simulink model "FOC_ADRC1"  (R2021b)
settings: Solver=ode3  StartTime=0.0  StopTime=0.6
InitFcn:
  | Ld=0.2e-3;
  | Lq=0.47e-3;
  | flux=0.062;
  | Rs=0.025;
  | b=1600;
libraries: simulink x2, spsDCVoltageSourceLib x1, spsPermanentMagnetSynchronousMachineLib x1, spsUniversalBridgeLib x1, spspowerguiLib x1
settings Model: SimulationMode=accelerator  Creator=lzy  LastModifiedBy=乐无安
settings SolverCC: AlgebraicLoopSolver=LineSearch
settings DebuggingCC: SFMachineParentedDataDiag=warning

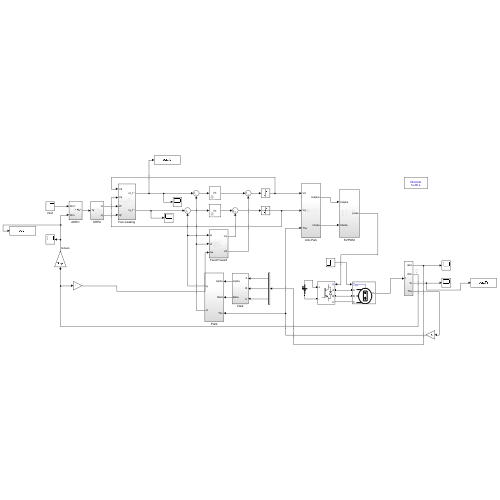
[thumbnail: Simulink's stored preview of the top-level diagram]
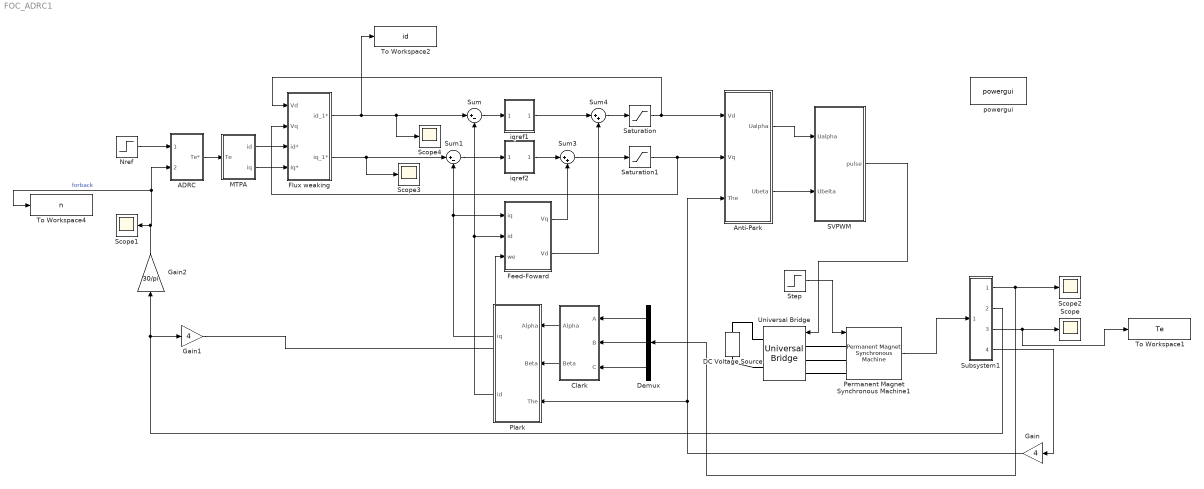
== system FOC_ADRC1 ==
  ADRC : Subsystem
  Anti-Park : Subsystem
  Clark : Subsystem
  DC Voltage Source : spsDCVoltageSourceLib/DC Voltage Source  Amplitude=192  Measurements=None
  Demux : Demux  Outputs=3
  Feed-Foward : Subsystem
  Flux weaking : Subsystem
  Gain : Gain  Gain=4
  Gain1 : Gain  Gain=4
  Gain2 : Gain  Gain=30/pi
  MTPA : Subsystem
  Nref : Step  Time=0.2  Before=3500  After=5500  SampleTime=0
  Permanent Magnet Synchronous Machine1 : spsPermanentMagnetSynchronousMachineLib/Permanent Magnet Synchronous Machine  NbPhases=3  FluxDistribution=Sinusoidal  RotorType=Salient-pole  MechanicalLoad=Torque Tm  PresetModel=No  ShowDetailedParameters=on  MeasurementBus=off  Resistance=0.029  Inductance=8.5e-3  dqInductances=[0.2e-3 0.47e-3]  La=0.015  MachineConstant=Flux linkage established by magnets (V.s)  Flux=0.062  VoltageCst=44.9822  TorqueCst=0.372  Flat=120  Mechanical=[1e-2 0 4]  PolePairs=3  InitialConditions=[0,0, 0,0]  InitialConditions5ph=[0 0 0 0 0 0]  RefAngle=Aligned with phase A axis (original Park)  IterativeDiscreteModel=Trapezoidal non iterative  TsBlock=-1  TsPowergui=0
  Plark : Subsystem
  SVPWM : Subsystem
  Saturation : Saturate  UpperLimit=192/1.732  LowerLimit=-192/1.732
  Saturation1 : Saturate  UpperLimit=192/1.732  LowerLimit=-192/1.732
  Scope{,1..4} (5 alike) : Scope
  Step : Step  Time=0.4  After=13  SampleTime=0
  Subsystem1 : Subsystem
  Sum : Sum  Inputs=|+-
  Sum1 : Sum  Inputs=|+-
  Sum3 : Sum  Inputs=|++
  Sum4 : Sum  Inputs=|++
  To Workspace1 : ToWorkspace  VariableName=Te  SampleTime=-1
      settings: Save2DSignal=2-D array (concatenate along first dimension)
  To Workspace2 : ToWorkspace  VariableName=id  SampleTime=-1
      settings: Save2DSignal=2-D array (concatenate along first dimension)
  To Workspace4 : ToWorkspace  VariableName=n  SampleTime=-1
      settings: Save2DSignal=2-D array (concatenate along first dimension)
  Universal Bridge : spsUniversalBridgeLib/Universal Bridge  Arms=3  SnubberResistance=1e5  SnubberCapacitance=inf  Device=IGBT / Diodes  Ron=1e-3  Lon=0  ForwardVoltages="[  0  0  ]"  ForwardVoltage=0  GTOparameters=[ 10e-6 , 20e-6 ]  IGBTparameters=[ 1e-6 , 2e-6 ]  Measurements=None  Measurements_2=None  converterType=Rectifier
  iqref1 : Subsystem  mask(PI Controller){I=60, P=40, sat=[-192/1.732,192/1.732]}
      mask prompts: I "Integral"; P "Proportional:"; sat "Minimum and maximum outputs:"
      mask init:
      | min=sat(1);max=sat(2);
      mask Display: disp('PI')
  iqref2 : Subsystem  mask(PI Controller){I=60, P=20, sat=[-192/1.732,192/1.732]}
      mask prompts: I "Integral"; P "Proportional:"; sat "Minimum and maximum outputs:"
      mask init:
      | min=sat(1);max=sat(2);
      mask Display: disp('PI')
  powergui : spspowerguiLib/powergui  Priority=1  SimulationMode=Discrete  SampleTime=10e-7  frequency=60  Iterations=50  frequencyindice=0  Pbase=100e6  ErrMax=1e-4  UnitsV=kV  UnitsW=MW  buscounter=0  FunctionMessages=off  echomessages=off  EnableUseOfTLC=off  CurrentSourceSwitches=off  DisableSnubberDevices=off  DisableRonSwitches=off  DisableVfSwitches=off  DisplayEquations=off  AutomaticDiscreteSolvers=off  SolverType=Tustin/Backward Euler (TBE)  Interpol=off  ExternalGateDelay=off  methode=off  Ts=100  x0status=blocks  SPID=on  SwTol=0  HookPort=off  NonlinearTolerance=1e-4  nMaxIteration=100  ContinueOnMaxIteration=off  RestoreLinks=warning  ResistiveCurrentMeasurement=off  Frange=[0:2:500]  Ylog=off  Xlog=on  ShowGrid=off  save=off  variable=ZData  structure=0  ZoomFFT=off  StartTime=0.0  cycles=1  DisplayStyle=1  fundamental=60  FreqAxis=off  MaxFrequency=1000  frequencyindicesteady=1  RmsSteady=1  display=off
  wires:
  Subsystem1/1(iabc) -> Scope2/1, Demux/1
  Sum/1 -> iqref1/1(In_1)
  Sum1/1 -> iqref2/1(In_1)
  Subsystem1/3(Te) -> To Workspace1/1, Scope/1
  Subsystem1/2(Wm) -> Gain1/1, Gain2/1
  Permanent Magnet Synchronous Machine1/1 -> Subsystem1/1(In1)
  Flux weaking/2(iq_1*) -> Scope3/1, Sum1/1
  Sum4/1 -> Saturation/1
  Sum3/1 -> Saturation1/1
  iqref2/1(Out_1) -> Sum3/1
  iqref1/1(Out_1) -> Sum4/1
  MTPA/1(id) -> Flux weaking/3(id*)
  Gain2/1 -> Scope1/1, To Workspace4/1, ADRC/2(Wm)  "forback"
  Step/1 -> Permanent Magnet Synchronous Machine1/1
  Clark/1(Alpha) -> Plark/1(Alpha)
  Demux/1 -> Clark/1(A)
  Demux/2 -> Clark/2(B)
  Demux/3 -> Clark/3(C)
  SVPWM/1(pulse) -> Universal Bridge/1
  ADRC/1(Te*) -> MTPA/1(Te)
  Anti-Park/1(Ualpha) -> SVPWM/1(Ualpha)
  Anti-Park/2(Ubeta) -> SVPWM/2(Ubelta)
  Subsystem1/4(The) -> Gain/1
  Clark/2(Beta) -> Plark/2(Beta)
  Plark/2(id) -> Feed-Foward/2(id), Sum/2
  Plark/1(iq) -> Feed-Foward/1(iq), Sum1/2
  Flux weaking/1(id_1*) -> To Workspace2/1, Scope4/1, Sum/1
  Gain1/1 -> Feed-Foward/3(we)
  Feed-Foward/1(Vq) -> Sum3/2
  Feed-Foward/2(Vd) -> Sum4/2
  Gain/1 -> Anti-Park/3(The), Plark/3(The)
  MTPA/2(iq) -> Flux weaking/4(Iq*)
  Nref/1 -> ADRC/1(Wm*)
  Saturation1/1 -> Flux weaking/2(Vq), Anti-Park/2(Vq)
  Saturation/1 -> Flux weaking/1(Vd), Anti-Park/1(Vd)
  connections:
  Universal Bridge/RConn1 -- DC Voltage Source/RConn1
  Universal Bridge/RConn2 -- DC Voltage Source/LConn1
  Universal Bridge/LConn3 -- Permanent Magnet Synchronous Machine1/LConn3
  Permanent Magnet Synchronous Machine1/LConn2 -- Universal Bridge/LConn2
  Permanent Magnet Synchronous Machine1/LConn1 -- Universal Bridge/LConn1

== system FOC_ADRC1/ADRC ==
  Wm* : Inport
  Wm : Inport  Port=2
  1/b : Gain  Gain=1/2000
  ESO : Subsystem
  Nlsef : Subsystem
  Saturation : Saturate  UpperLimit=72  LowerLimit=-72
  Sum : Sum  Inputs=|+-
  TD : Subsystem
  b : Gain  Gain=b
  Te* : Outport
  wires:
  Wm/1 -> ESO/2(Wm)
  Wm*/1 -> TD/1(Wm*)
  b/1 -> ESO/1(bu)
  TD/1(Z11) -> Nlsef/1(Z11)
  1/b/1 -> Sum/2
  Nlsef/1(u0) -> Sum/1
  Sum/1 -> Saturation/1, b/1
  Saturation/1 -> Te*/1
  ESO/2(Z21) -> Nlsef/2(Z21)
  ESO/1(Z22) -> 1/b/1

== system FOC_ADRC1/Anti-Park ==
  Vd : Inport
  Vq : Inport  Port=2
  The : Inport  Port=3
  Fcn : Fcn  Expr=cos(u[1])*u[2]-sin(u[1])*u[3]
  Fcn1 : Fcn  Expr=sin(u[1])*u[2]+cos(u[1])*u[3]
  Mux1 : Mux  Inputs=3
  Ualpha : Outport  VectorParamsAs1DForOutWhenUnconnected=off
  Ubeta : Outport  Port=2  VectorParamsAs1DForOutWhenUnconnected=off
  wires:
  Vd/1 -> Mux1/2
  The/1 -> Mux1/1
  Fcn1/1 -> Ubeta/1
  Vq/1 -> Mux1/3
  Fcn/1 -> Ualpha/1
  Mux1/1 -> Fcn/1, Fcn1/1

== system FOC_ADRC1/Clark ==
  A : Inport
  B : Inport  Port=2
  C : Inport  Port=3
  Mux : Mux  Inputs=3
  alpha : Fcn  Expr=(u(1)-0.5*(u(2)+u(3)))*2/3
  beta : Fcn  Expr=sqrt(3)/2*(u(2)-u(3))*2/3
  Alpha : Outport  VectorParamsAs1DForOutWhenUnconnected=off
  Beta : Outport  Port=2  VectorParamsAs1DForOutWhenUnconnected=off
  wires:
  B/1 -> Mux/2
  C/1 -> Mux/3
  beta/1 -> Beta/1
  A/1 -> Mux/1
  Mux/1 -> beta/1, alpha/1
  alpha/1 -> Alpha/1

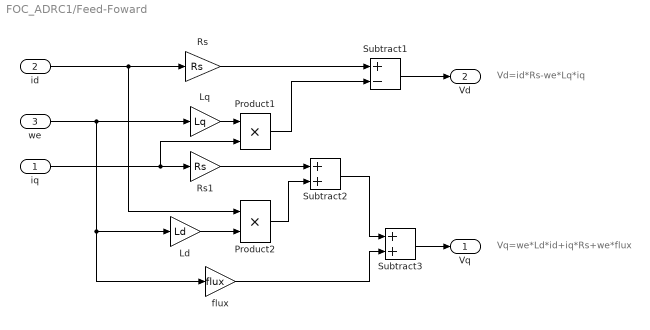
== system FOC_ADRC1/Feed-Foward ==
  note: Vd=id*Rs-we*Lq*iq
  note: Vq=we*Ld*id+iq*Rs+we*flux
  iq : Inport
  id : Inport  Port=2
  we : Inport  Port=3
  Ld : Gain  Gain=Ld
  Lq : Gain  Gain=Lq
  Product1 : Product  RndMeth=Zero
  Product2 : Product  RndMeth=Zero
  Rs : Gain  Gain=Rs
  Rs1 : Gain  Gain=Rs
  Subtract1 : Sum  Inputs=+-
  Subtract2 : Sum
  Subtract3 : Sum
  flux : Gain  Gain=flux
  Vq : Outport  VectorParamsAs1DForOutWhenUnconnected=off
  Vd : Outport  Port=2  VectorParamsAs1DForOutWhenUnconnected=off
  wires:
  Subtract2/1 -> Subtract3/1
  iq/1 -> Rs1/1, Product1/2
  we/1 -> Lq/1, Ld/1, flux/1
  flux/1 -> Subtract3/2
  Product2/1 -> Subtract2/2
  id/1 -> Rs/1, Product2/1
  Lq/1 -> Product1/1
  Product1/1 -> Subtract1/2
  Subtract1/1 -> Vd/1
  Rs/1 -> Subtract1/1
  Rs1/1 -> Subtract2/1
  Ld/1 -> Product2/2
  Subtract3/1 -> Vq/1

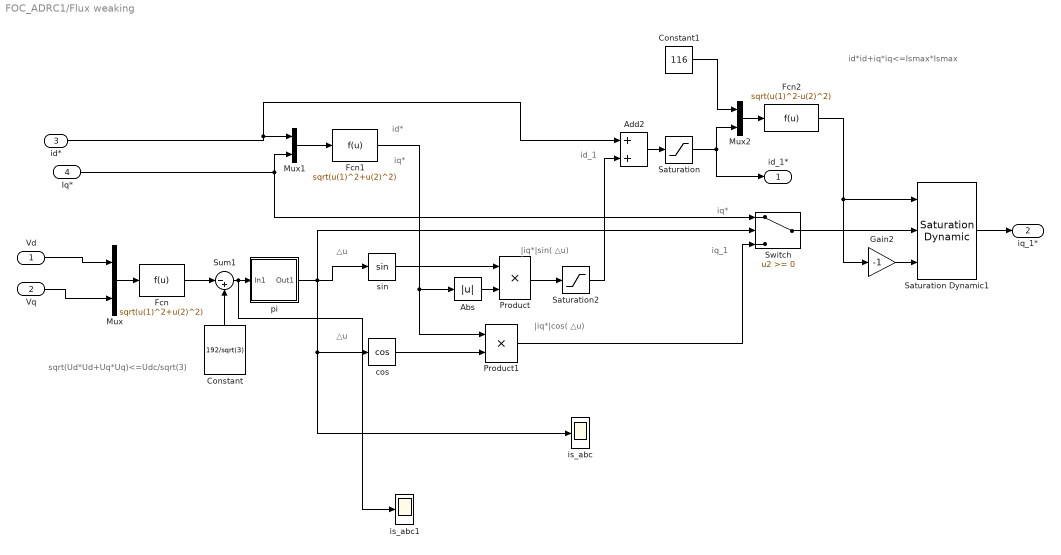
== system FOC_ADRC1/Flux weaking ==
  note: |iq*|cos( △u)
  note: iq*
  note: id*id+iq*iq<=Ismax*Ismax
  note: |iq*|sin( △u)
  note: sqrt(Ud*Ud+Uq*Uq)<=Udc/sqrt(3)
  note: id*
  note: △u
  note: △u
  note: iq*
  note: id_1
  note: iq_1
  Vd : Inport
  Vq : Inport  Port=2
  id* : Inport  Port=3
  Iq* : Inport  Port=4
  Abs : Abs
  Add2 : Sum  OutDataTypeStr=Inherit: Same as first input
  Constant : Constant  Value=192/sqrt(3)  SampleTime=-1
  Constant1 : Constant  Value=116  SampleTime=-1
  Fcn : Fcn  Expr=sqrt(u(1)^2+u(2)^2)
  Fcn1 : Fcn  Expr=sqrt(u(1)^2+u(2)^2)
  Fcn2 : Fcn  Expr=sqrt(u(1)^2-u(2)^2)
  Gain2 : Gain  Gain=-1
  Mux : Mux  Inputs=2
  Mux1 : Mux  Inputs=2
  Mux2 : Mux  Inputs=2
  Product : Product  RndMeth=Zero
  Product1 : Product  RndMeth=Zero
  Saturation : Saturate  UpperLimit=100  LowerLimit=-100
  Saturation Dynamic1 : simulink/Discontinuities/Saturation Dynamic  OutMin=[]  OutMax=[]  OutDataTypeStr=Inherit: Same as second input  OutDataType=fixdt(1, 16)  OutScaling=2^-10  DoSatur=off
  Saturation2 : Saturate  UpperLimit=0  LowerLimit=-flux/Ld
  Sum1 : Sum  Inputs=|-+
  Switch : Switch
  cos : Trigonometry  Operator=cos
  is_abc : Scope
  is_abc1 : Scope
  pi : Subsystem
  sin : Trigonometry
  id_1* : Outport  VectorParamsAs1DForOutWhenUnconnected=off
  iq_1* : Outport  Port=2  VectorParamsAs1DForOutWhenUnconnected=off
  wires:
  Vd/1 -> Mux/1
  pi/1(Out1) -> cos/1, is_abc/1, Switch/2, sin/1
  Constant/1 -> Sum1/2
  Product1/1 -> Switch/3
  cos/1 -> Product1/2
  Vq/1 -> Mux/2
  Saturation/1 -> Mux2/2, id_1*/1
  Product/1 -> Saturation2/1
  Mux/1 -> Fcn/1
  Mux2/1 -> Fcn2/1
  Constant1/1 -> Mux2/1
  sin/1 -> Product/1
  Fcn/1 -> Sum1/1
  Abs/1 -> Product/2
  Saturation Dynamic1/1 -> iq_1*/1
  Fcn2/1 -> Saturation Dynamic1/1, Gain2/1
  Switch/1 -> Saturation Dynamic1/2
  Gain2/1 -> Saturation Dynamic1/3
  Sum1/1 -> is_abc1/1, pi/1(In1)
  Add2/1 -> Saturation/1
  Saturation2/1 -> Add2/2
  Iq*/1 -> Mux1/2, Switch/1
  id*/1 -> Add2/1, Mux1/1
  Mux1/1 -> Fcn1/1
  Fcn1/1 -> Abs/1, Product1/1

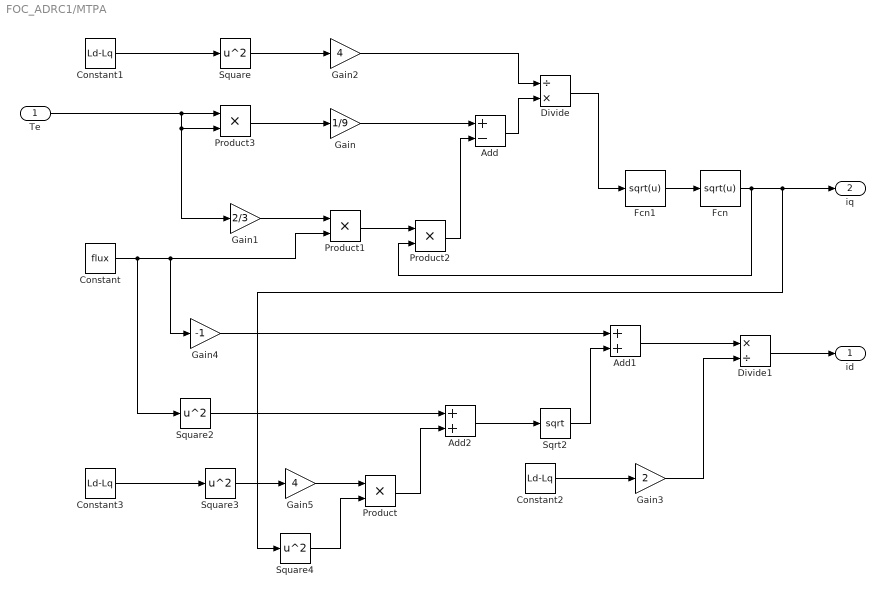
== system FOC_ADRC1/MTPA ==
  Te : Inport
  Add : Sum  Inputs=+-
  Add1 : Sum
  Add2 : Sum
  Constant : Constant  Value=flux
  Constant1 : Constant  Value=Ld-Lq
  Constant2 : Constant  Value=Ld-Lq
  Constant3 : Constant  Value=Ld-Lq
  Divide : Product  Inputs=/*
  Divide1 : Product  Inputs=*/
  Fcn : Fcn  Expr=sqrt(u)
  Fcn1 : Fcn  Expr=sqrt(u)
  Gain : Gain  Gain=1/9
  Gain1 : Gain  Gain=2/3
  Gain2 : Gain  Gain=4
  Gain3 : Gain  Gain=2
  Gain4 : Gain  Gain=-1
  Gain5 : Gain  Gain=4
  Product{,1..3} (4 alike) : Product
  Sqrt2 : Sqrt  SaturateOnIntegerOverflow=on
  Square{,2..4} (4 alike) : Math  Operator=square  SaturateOnIntegerOverflow=on
  id : Outport
  iq : Outport  Port=2
  wires:
  Gain/1 -> Add/1
  Gain1/1 -> Product1/1
  Constant/1 -> Square2/1, Gain4/1, Product1/2
  Product1/1 -> Product2/1
  Product3/1 -> Gain/1
  Constant1/1 -> Square/1
  Square/1 -> Gain2/1
  Fcn/1 -> iq/1, Square4/1, Product2/2
  Product2/1 -> Add/2
  Add/1 -> Divide/2
  Gain2/1 -> Divide/1
  Constant2/1 -> Gain3/1
  Gain4/1 -> Add1/1
  Square2/1 -> Add2/1
  Constant3/1 -> Square3/1
  Square3/1 -> Gain5/1
  Gain5/1 -> Product/1
  Square4/1 -> Product/2
  Product/1 -> Add2/2
  Add2/1 -> Sqrt2/1
  Sqrt2/1 -> Add1/2
  Divide1/1 -> id/1
  Add1/1 -> Divide1/1
  Gain3/1 -> Divide1/2
  Te/1 -> Gain1/1, Product3/2, Product3/1
  Fcn1/1 -> Fcn/1
  Divide/1 -> Fcn1/1

== system FOC_ADRC1/Plark ==
  Alpha : Inport
  Beta : Inport  Port=2
  The : Inport  Port=3
  Mux : Mux  Inputs=3
  d : Fcn  Expr=u(1)*cos(u(3))+u(2)*sin(u(3))
  q : Fcn  Expr=-u(1)*sin(u(3))+u(2)*cos(u(3))
  iq : Outport  VectorParamsAs1DForOutWhenUnconnected=off
  id : Outport  Port=2  VectorParamsAs1DForOutWhenUnconnected=off
  wires:
  Alpha/1 -> Mux/1
  The/1 -> Mux/3
  Beta/1 -> Mux/2
  d/1 -> id/1
  Mux/1 -> q/1, d/1
  q/1 -> iq/1

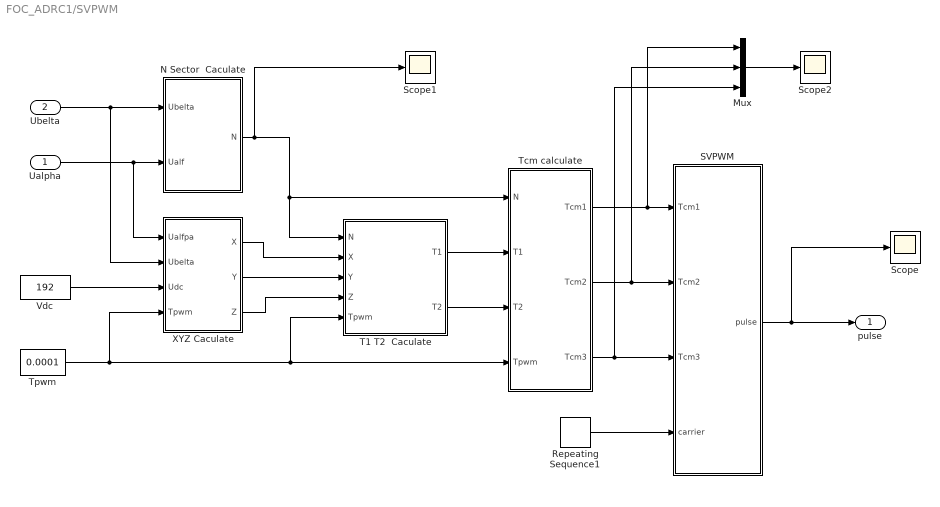
== system FOC_ADRC1/SVPWM ==
  Ualpha : Inport
  Ubelta : Inport  Port=2
  Mux : Mux  Inputs=3
  N Sector  Caculate : Subsystem  TreatAsAtomicUnit=on
  Repeating Sequence1 : simulink/Sources/Repeating Sequence  rep_seq_t=[0 0.00005 0.0001]  rep_seq_y=[0 0.00005 0]
  SVPWM : Subsystem  TreatAsAtomicUnit=on
  Scope : Scope
  Scope1 : Scope
  Scope2 : Scope
  T1 T2  Caculate : Subsystem  TreatAsAtomicUnit=on
  Tcm calculate : Subsystem  TreatAsAtomicUnit=on
  Tpwm : Constant  Value=0.0001
  Vdc : Constant  Value=192
  XYZ Caculate : Subsystem  TreatAsAtomicUnit=on
  pulse : Outport  VectorParamsAs1DForOutWhenUnconnected=off
  wires:
  Ualpha/1 -> N Sector  Caculate/2(Ualf), XYZ Caculate/1(Ualfpa)
  Tcm calculate/2(Tcm2) -> Mux/2, SVPWM/2(Tcm2)
  T1 T2  Caculate/1(T1) -> Tcm calculate/2(T1)
  Tcm calculate/3(Tcm3) -> Mux/3, SVPWM/3(Tcm3)
  Tcm calculate/1(Tcm1) -> Mux/1, SVPWM/1(Tcm1)
  N Sector  Caculate/1(N) -> Scope1/1, T1 T2  Caculate/1(N), Tcm calculate/1(N)
  Repeating Sequence1/1 -> SVPWM/4(carrier)
  Tpwm/1 -> XYZ Caculate/4(Tpwm), T1 T2  Caculate/5(Tpwm), Tcm calculate/4(Tpwm)
  SVPWM/1(pulse) -> Scope/1, pulse/1
  T1 T2  Caculate/2(T2) -> Tcm calculate/3(T2)
  XYZ Caculate/1(X) -> T1 T2  Caculate/2(X)
  Ubelta/1 -> N Sector  Caculate/1(Ubelta), XYZ Caculate/2(Ubelta)
  Vdc/1 -> XYZ Caculate/3(Udc)
  XYZ Caculate/2(Y) -> T1 T2  Caculate/3(Y)
  XYZ Caculate/3(Z) -> T1 T2  Caculate/4(Z)
  Mux/1 -> Scope2/1

== system FOC_ADRC1/Subsystem1 ==
  In1 : Inport
  Bus Selector1 : BusSelector  OutputSignals=Stator current is_a (A),Stator current is_b (A),Stator current is_c (A)
  Bus Selector2 : BusSelector  OutputSignals=Rotor speed wm (rad/s),Rotor angle thetam (rad),Electromagnetic torque Te (N*m)
  Mux : Mux  Inputs=3
  iabc : Outport
  Wm : Outport  Port=2
  Te : Outport  Port=3
  The : Outport  Port=4
  wires:
  In1/1 -> Bus Selector2/1, Bus Selector1/1
  Bus Selector1/3 -> Mux/3  "<Stator current is_c (A)>"
  Bus Selector1/2 -> Mux/2  "<Stator current is_b (A)>"
  Bus Selector1/1 -> Mux/1  "<Stator current is_a (A)>"
  Mux/1 -> iabc/1
  Bus Selector2/2 -> The/1  "<Rotor angle thetam (rad)>"
  Bus Selector2/1 -> Wm/1  "<Rotor speed wm (rad/s)>"
  Bus Selector2/3 -> Te/1  "<Electromagnetic torque Te (N*m)>"

== system FOC_ADRC1/iqref1 ==
  In_1 : Inport
  Integrator1 : Integrator  LimitOutput=on  UpperSaturationLimit=max  LowerSaturationLimit=min
  Proportional : Gain  Gain=P  SaturateOnIntegerOverflow=on  OutDataTypeStr=Inherit: Same as input  ParamDataTypeStr=Inherit: Same as input
  Proportional1 : Gain  Gain=I  SaturateOnIntegerOverflow=on  OutDataTypeStr=Inherit: Same as input  ParamDataTypeStr=Inherit: Same as input
  Saturation : Saturate  UpperLimit=max  LowerLimit=min
  Sum : Sum  InputSameDT=on  SaturateOnIntegerOverflow=on  OutDataTypeStr=Inherit: Same as first input
  Out_1 : Outport  InitialOutput=0  VectorParamsAs1DForOutWhenUnconnected=off
  wires:
  Saturation/1 -> Out_1/1
  Sum/1 -> Saturation/1
  Proportional/1 -> Sum/1
  In_1/1 -> Proportional1/1, Proportional/1
  Integrator1/1 -> Sum/2
  Proportional1/1 -> Integrator1/1

== system FOC_ADRC1/iqref2 ==
  In_1 : Inport
  Integrator1 : Integrator  LimitOutput=on  UpperSaturationLimit=max  LowerSaturationLimit=min
  Proportional : Gain  Gain=P  SaturateOnIntegerOverflow=on  OutDataTypeStr=Inherit: Same as input  ParamDataTypeStr=Inherit: Same as input
  Proportional1 : Gain  Gain=I  SaturateOnIntegerOverflow=on  OutDataTypeStr=Inherit: Same as input  ParamDataTypeStr=Inherit: Same as input
  Saturation : Saturate  UpperLimit=max  LowerLimit=min
  Sum : Sum  InputSameDT=on  SaturateOnIntegerOverflow=on  OutDataTypeStr=Inherit: Same as first input
  Out_1 : Outport  InitialOutput=0  VectorParamsAs1DForOutWhenUnconnected=off
  wires:
  In_1/1 -> Proportional1/1, Proportional/1
  Proportional/1 -> Sum/1
  Sum/1 -> Saturation/1
  Saturation/1 -> Out_1/1
  Integrator1/1 -> Sum/2
  Proportional1/1 -> Integrator1/1

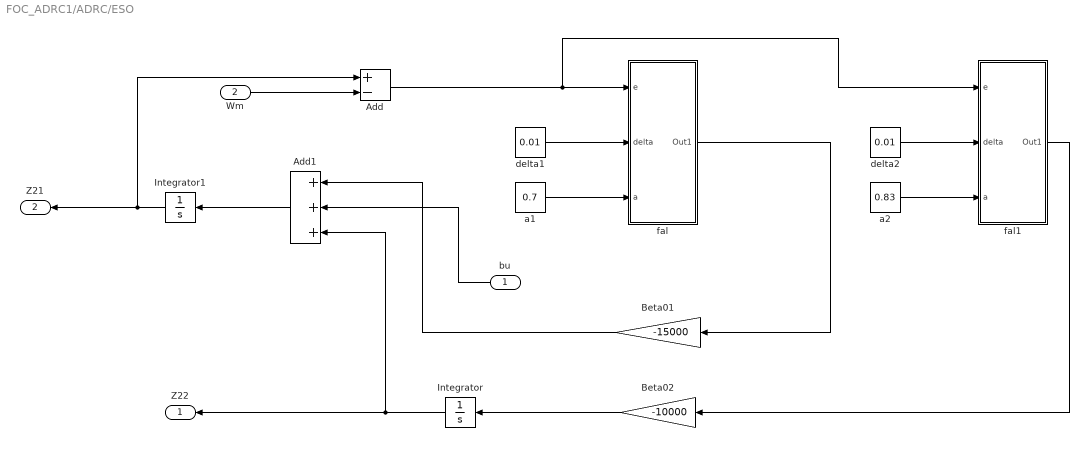
== system FOC_ADRC1/ADRC/ESO ==
  bu : Inport
  Wm : Inport  Port=2
  Add : Sum  Inputs=+-
  Add1 : Sum  Inputs=+++
  Beta01 : Gain  Gain=-15000
  Beta02 : Gain  Gain=-10000
  Integrator : Integrator
  Integrator1 : Integrator
  a1 : Constant  Value=0.7
  a2 : Constant  Value=0.83
  delta1 : Constant  Value=0.01
  delta2 : Constant  Value=0.01
  fal : Subsystem
  fal1 : Subsystem
  Z22 : Outport
  Z21 : Outport  Port=2
  wires:
  Add/1 -> fal1/1(e), fal/1(e)
  delta1/1 -> fal/2(delta)
  a1/1 -> fal/3(a)
  delta2/1 -> fal1/2(delta)
  a2/1 -> fal1/3(a)
  fal/1(Out1) -> Beta01/1
  fal1/1(Out1) -> Beta02/1
  Beta02/1 -> Integrator/1
  Integrator/1 -> Z22/1, Add1/3
  Beta01/1 -> Add1/1
  bu/1 -> Add1/2
  Add1/1 -> Integrator1/1
  Integrator1/1 -> Z21/1, Add/1
  Wm/1 -> Add/2

== system FOC_ADRC1/ADRC/Nlsef ==
  Z11 : Inport
  Z21 : Inport  Port=2
  Add : Sum  Inputs=+-
  Constant : Constant  Value=0.01
  Constant1 : Constant  Value=0.9
  fal : Subsystem
  k : Gain  Gain=980
  u0 : Outport
  wires:
  fal/1(Out1) -> k/1
  Z21/1 -> Add/2
  Z11/1 -> Add/1
  Add/1 -> fal/1(e)
  k/1 -> u0/1
  Constant/1 -> fal/2(delta)
  Constant1/1 -> fal/3(a)

== system FOC_ADRC1/ADRC/TD ==
  Wm* : Inport
  Add : Sum  Inputs=-+
  Integrator : Integrator
  a0 : Constant  Value=0.4
  delta0 : Constant  Value=0.01
  fal : Subsystem
  r : Gain  Gain=-3000
  Z11 : Outport
  wires:
  fal/1(Out1) -> r/1
  r/1 -> Integrator/1
  Integrator/1 -> Add/2, Z11/1
  delta0/1 -> fal/2(delta)
  a0/1 -> fal/3(a)
  Wm*/1 -> Add/1
  Add/1 -> fal/1(e)

== system FOC_ADRC1/Flux weaking/pi ==
  In1 : Inport
  Gain2 : Gain  Gain=9
  Integrator : Integrator  LimitOutput=on  UpperSaturationLimit=0  LowerSaturationLimit=-1.57
  Out1 : Outport  VectorParamsAs1DForOutWhenUnconnected=off
  wires:
  Gain2/1 -> Integrator/1
  In1/1 -> Gain2/1
  Integrator/1 -> Out1/1

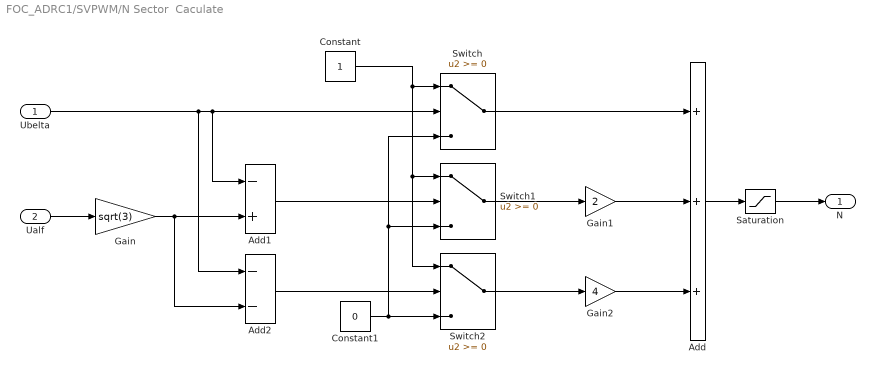
== system FOC_ADRC1/SVPWM/N Sector  Caculate ==
  Ubelta : Inport
  Ualf : Inport  Port=2
  Add : Sum  Inputs=+++
  Add1 : Sum  Inputs=-+
  Add2 : Sum  Inputs=--
  Constant : Constant
  Constant1 : Constant  Value=0
  Gain : Gain  Gain=sqrt(3)
  Gain1 : Gain  Gain=2
  Gain2 : Gain  Gain=4
  Saturation : Saturate  UpperLimit=6  LowerLimit=1
  Switch : Switch
  Switch1 : Switch
  Switch2 : Switch
  N : Outport  VectorParamsAs1DForOutWhenUnconnected=off
  wires:
  Saturation/1 -> N/1
  Add/1 -> Saturation/1
  Gain2/1 -> Add/3
  Switch2/1 -> Gain2/1
  Add2/1 -> Switch2/2
  Gain1/1 -> Add/2
  Switch1/1 -> Gain1/1
  Add1/1 -> Switch1/2
  Gain/1 -> Add2/2, Add1/2
  Ualf/1 -> Gain/1
  Switch/1 -> Add/1
  Constant1/1 -> Switch/3, Switch1/3, Switch2/3
  Constant/1 -> Switch/1, Switch1/1, Switch2/1
  Ubelta/1 -> Add2/1, Add1/1, Switch/2

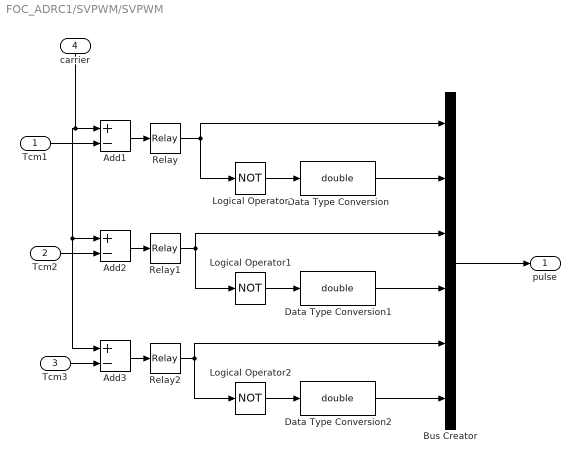
== system FOC_ADRC1/SVPWM/SVPWM ==
  Tcm1 : Inport
  Tcm2 : Inport  Port=2
  Tcm3 : Inport  Port=3
  carrier : Inport  Port=4
  Add1 : Sum  Inputs=+-
  Add2 : Sum  Inputs=+-
  Add3 : Sum  Inputs=+-
  Bus Creator : BusCreator  Inputs=6
  Data Type Conversion : DataTypeConversion  OutDataTypeStr=double
  Data Type Conversion1 : DataTypeConversion  OutDataTypeStr=double
  Data Type Conversion2 : DataTypeConversion  OutDataTypeStr=double
  Logical Operator : Logic  Operator=NOT  AllPortsSameDT=off  OutDataTypeStr=boolean
  Logical Operator1 : Logic  Operator=NOT  AllPortsSameDT=off  OutDataTypeStr=boolean
  Logical Operator2 : Logic  Operator=NOT  AllPortsSameDT=off  OutDataTypeStr=boolean
  Relay : Relay
  Relay1 : Relay
  Relay2 : Relay
  pulse : Outport  VectorParamsAs1DForOutWhenUnconnected=off
  wires:
  carrier/1 -> Add1/1, Add2/1, Add3/1
  Tcm2/1 -> Add2/2
  Tcm3/1 -> Add3/2
  Add3/1 -> Relay2/1
  Add2/1 -> Relay1/1
  Add1/1 -> Relay/1
  Tcm1/1 -> Add1/2
  Relay2/1 -> Logical Operator2/1, Bus Creator/5
  Relay/1 -> Logical Operator/1, Bus Creator/1
  Relay1/1 -> Logical Operator1/1, Bus Creator/3
  Data Type Conversion2/1 -> Bus Creator/6
  Logical Operator2/1 -> Data Type Conversion2/1
  Data Type Conversion1/1 -> Bus Creator/4
  Logical Operator1/1 -> Data Type Conversion1/1
  Data Type Conversion/1 -> Bus Creator/2
  Logical Operator/1 -> Data Type Conversion/1
  Bus Creator/1 -> pulse/1

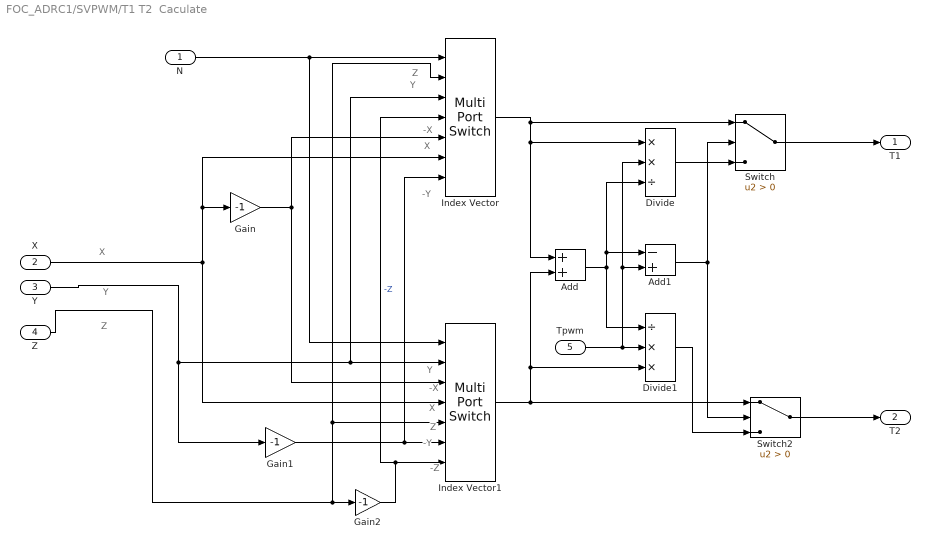
== system FOC_ADRC1/SVPWM/T1 T2  Caculate ==
  note: Z
  note: Y
  note: -X
  note: X
  note: -Y
  note: Y
  note: -X
  note: X
  note: Z
  note: -Y
  note: -Z
  note: X
  note: Y
  note: Z
  N : Inport
  X : Inport  Port=2
  Y : Inport  Port=3
  Z : Inport  Port=4
  Tpwm : Inport  Port=5
  Add : Sum
  Add1 : Sum  Inputs=-+
  Divide : Product  Inputs=**/
  Divide1 : Product  Inputs=/**
  Gain : Gain  Gain=-1
  Gain1 : Gain  Gain=-1
  Gain2 : Gain  Gain=-1
  Index Vector : MultiPortSwitch  Inputs=6
  Index Vector1 : MultiPortSwitch  Inputs=6
  Switch : Switch  Criteria=u2 > Threshold
  Switch2 : Switch  Criteria=u2 > Threshold
  T1 : Outport  VectorParamsAs1DForOutWhenUnconnected=off
  T2 : Outport  Port=2  VectorParamsAs1DForOutWhenUnconnected=off
  wires:
  Switch2/1 -> T2/1
  Divide1/1 -> Switch2/3
  Switch/1 -> T1/1
  Add1/1 -> Switch/2, Switch2/2
  Add/1 -> Divide1/1, Divide/3, Add1/1
  Tpwm/1 -> Divide1/2, Divide/2, Add1/2
  Divide/1 -> Switch/3
  Index Vector1/1 -> Switch2/1, Add/2, Divide1/3
  Index Vector/1 -> Switch/1, Divide/1, Add/1
  Gain1/1 -> Index Vector/7, Index Vector1/6
  Gain2/1 -> Index Vector/4, Index Vector1/7  "-Z"
  Gain/1 -> Index Vector/5, Index Vector1/3
  Y/1 -> Gain1/1, Index Vector/3, Index Vector1/2
  X/1 -> Index Vector1/4, Index Vector/6, Gain/1
  Z/1 -> Index Vector/2, Index Vector1/5, Gain2/1
  N/1 -> Index Vector1/1, Index Vector/1

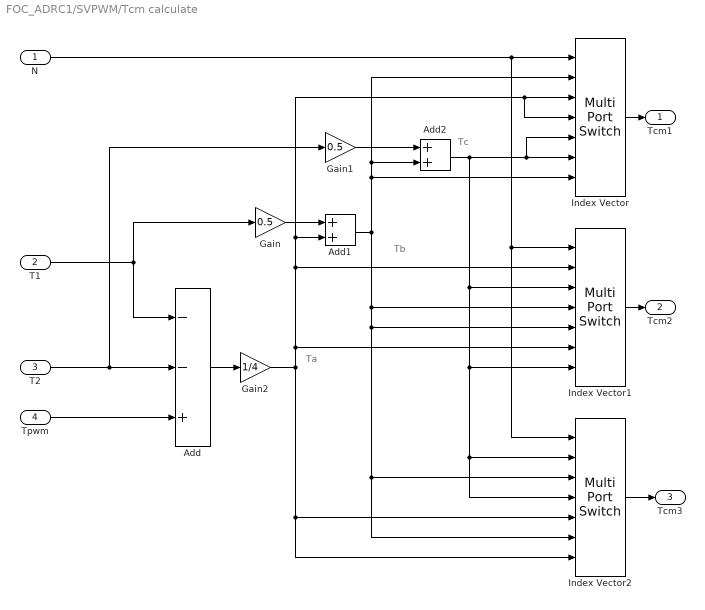
== system FOC_ADRC1/SVPWM/Tcm calculate ==
  note: Tc
  note: Tb
  note: Ta
  N : Inport
  T1 : Inport  Port=2
  T2 : Inport  Port=3
  Tpwm : Inport  Port=4
  Add : Sum  Inputs=--+
  Add1 : Sum
  Add2 : Sum
  Gain : Gain  Gain=0.5
  Gain1 : Gain  Gain=0.5
  Gain2 : Gain  Gain=1/4
  Index Vector : MultiPortSwitch  Inputs=6
  Index Vector1 : MultiPortSwitch  Inputs=6
  Index Vector2 : MultiPortSwitch  Inputs=6
  Tcm1 : Outport  VectorParamsAs1DForOutWhenUnconnected=off
  Tcm2 : Outport  Port=2  VectorParamsAs1DForOutWhenUnconnected=off
  Tcm3 : Outport  Port=3  VectorParamsAs1DForOutWhenUnconnected=off
  wires:
  Index Vector2/1 -> Tcm3/1
  N/1 -> Index Vector/1, Index Vector1/1, Index Vector2/1
  Add2/1 -> Index Vector/5, Index Vector/6, Index Vector1/3, Index Vector1/7, Index Vector2/2, Index Vector2/4
  Gain1/1 -> Add2/1
  Add1/1 -> Add2/2, Index Vector/2, Index Vector/7, Index Vector1/4, Index Vector1/5, Index Vector2/3, Index Vector2/6
  Gain2/1 -> Index Vector2/5, Index Vector2/7, Add1/2, Index Vector/3, Index Vector/4, Index Vector1/2, Index Vector1/6
  Gain/1 -> Add1/1
  Add/1 -> Gain2/1
  Tpwm/1 -> Add/3
  T2/1 -> Add/2, Gain1/1
  T1/1 -> Add/1, Gain/1
  Index Vector/1 -> Tcm1/1
  Index Vector1/1 -> Tcm2/1

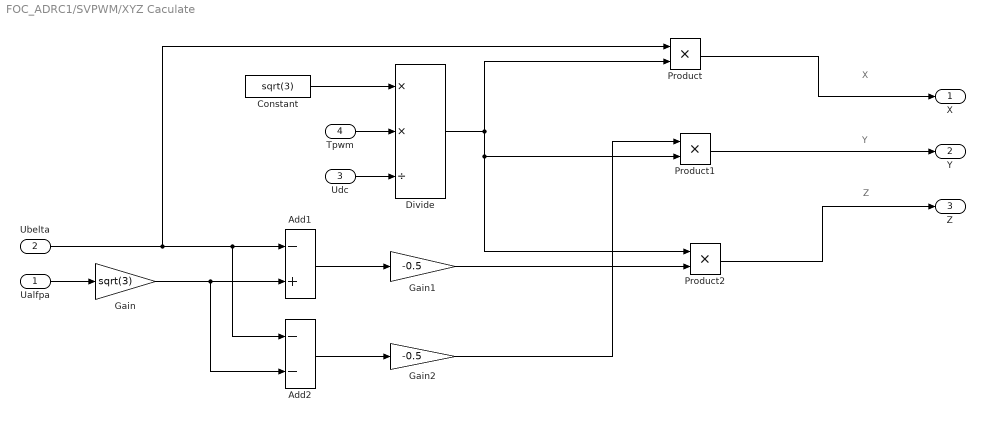
== system FOC_ADRC1/SVPWM/XYZ Caculate ==
  note: X
  note: Y
  note: Z
  Ualfpa : Inport
  Ubelta : Inport  Port=2
  Udc : Inport  Port=3
  Tpwm : Inport  Port=4
  Add1 : Sum  Inputs=-+
  Add2 : Sum  Inputs=--
  Constant : Constant  Value=sqrt(3)
  Divide : Product  Inputs=**/
  Gain : Gain  Gain=sqrt(3)
  Gain1 : Gain  Gain=-0.5
  Gain2 : Gain  Gain=-0.5
  Product : Product
  Product1 : Product
  Product2 : Product
  X : Outport  VectorParamsAs1DForOutWhenUnconnected=off
  Y : Outport  Port=2  VectorParamsAs1DForOutWhenUnconnected=off
  Z : Outport  Port=3  VectorParamsAs1DForOutWhenUnconnected=off
  wires:
  Gain2/1 -> Product1/1
  Add2/1 -> Gain2/1
  Add1/1 -> Gain1/1
  Gain/1 -> Add2/2, Add1/2
  Ualfpa/1 -> Gain/1
  Ubelta/1 -> Add2/1, Add1/1, Product/1
  Gain1/1 -> Product2/2
  Product2/1 -> Z/1
  Divide/1 -> Product1/2, Product2/1, Product/2
  Product1/1 -> Y/1
  Product/1 -> X/1
  Udc/1 -> Divide/3
  Tpwm/1 -> Divide/2
  Constant/1 -> Divide/1

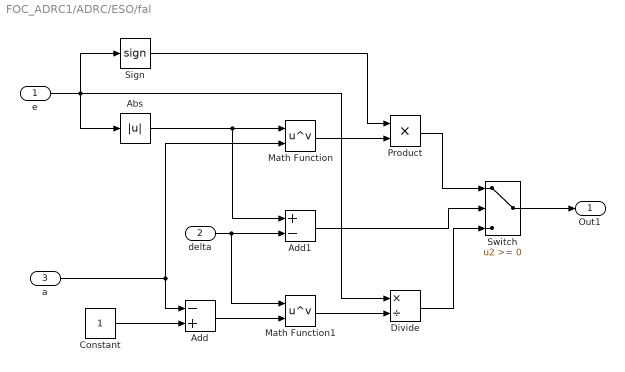
== system FOC_ADRC1/ADRC/ESO/fal ==
  e : Inport
  delta : Inport  Port=2
  a : Inport  Port=3
  Abs : Abs
  Add : Sum  Inputs=-+
  Add1 : Sum  Inputs=+-
  Constant : Constant
  Divide : Product  Inputs=*/
  Math Function : Math  Operator=pow  SignedPower=on  SaturateOnIntegerOverflow=on
  Math Function1 : Math  Operator=pow  SignedPower=on  SaturateOnIntegerOverflow=on
  Product : Product  RndMeth=Zero
  Sign : Signum
  Switch : Switch
  Out1 : Outport
  wires:
  a/1 -> Add/1, Math Function/2
  Constant/1 -> Add/2
  Abs/1 -> Math Function/1, Add1/1
  Math Function/1 -> Product/2
  Sign/1 -> Product/1
  delta/1 -> Add1/2, Math Function1/1
  Add1/1 -> Switch/2
  Product/1 -> Switch/1
  Add/1 -> Math Function1/2
  Math Function1/1 -> Divide/2
  Divide/1 -> Switch/3
  Switch/1 -> Out1/1
  e/1 -> Sign/1, Abs/1, Divide/1

== system FOC_ADRC1/ADRC/ESO/fal1 ==
  e : Inport
  delta : Inport  Port=2
  a : Inport  Port=3
  Abs : Abs
  Add : Sum  Inputs=-+
  Add1 : Sum  Inputs=+-
  Constant : Constant
  Divide : Product  Inputs=*/
  Math Function : Math  Operator=pow  SignedPower=on  SaturateOnIntegerOverflow=on
  Math Function1 : Math  Operator=pow  SignedPower=on  SaturateOnIntegerOverflow=on
  Product : Product  RndMeth=Zero
  Sign : Signum
  Switch : Switch
  Out1 : Outport
  wires:
  a/1 -> Add/1, Math Function/2
  Constant/1 -> Add/2
  Abs/1 -> Math Function/1, Add1/1
  Math Function/1 -> Product/2
  Sign/1 -> Product/1
  delta/1 -> Add1/2, Math Function1/1
  Add1/1 -> Switch/2
  Product/1 -> Switch/1
  Add/1 -> Math Function1/2
  Math Function1/1 -> Divide/2
  Divide/1 -> Switch/3
  Switch/1 -> Out1/1
  e/1 -> Sign/1, Abs/1, Divide/1

== system FOC_ADRC1/ADRC/Nlsef/fal ==
  e : Inport
  delta : Inport  Port=2
  a : Inport  Port=3
  Abs : Abs
  Add : Sum  Inputs=-+
  Add1 : Sum  Inputs=+-
  Constant : Constant
  Divide : Product  Inputs=*/
  Math Function : Math  Operator=pow  SignedPower=on  SaturateOnIntegerOverflow=on
  Math Function1 : Math  Operator=pow  SignedPower=on  SaturateOnIntegerOverflow=on
  Product : Product  RndMeth=Zero
  Sign : Signum
  Switch : Switch
  Out1 : Outport
  wires:
  a/1 -> Add/1, Math Function/2
  Constant/1 -> Add/2
  Abs/1 -> Math Function/1, Add1/1
  Math Function/1 -> Product/2
  Sign/1 -> Product/1
  delta/1 -> Add1/2, Math Function1/1
  Add1/1 -> Switch/2
  Product/1 -> Switch/1
  Add/1 -> Math Function1/2
  Math Function1/1 -> Divide/2
  Divide/1 -> Switch/3
  Switch/1 -> Out1/1
  e/1 -> Sign/1, Abs/1, Divide/1

== system FOC_ADRC1/ADRC/TD/fal ==
  e : Inport
  delta : Inport  Port=2
  a : Inport  Port=3
  Abs : Abs
  Add : Sum  Inputs=-+
  Add1 : Sum  Inputs=+-
  Constant : Constant
  Divide : Product  Inputs=*/
  Math Function : Math  Operator=pow  SignedPower=on  SaturateOnIntegerOverflow=on
  Math Function1 : Math  Operator=pow  SignedPower=on  SaturateOnIntegerOverflow=on
  Product : Product  RndMeth=Zero
  Sign : Signum
  Switch : Switch
  Out1 : Outport
  wires:
  a/1 -> Add/1, Math Function/2
  Constant/1 -> Add/2
  Abs/1 -> Math Function/1, Add1/1
  Math Function/1 -> Product/2
  Sign/1 -> Product/1
  delta/1 -> Add1/2, Math Function1/1
  Add1/1 -> Switch/2
  Product/1 -> Switch/1
  Add/1 -> Math Function1/2
  Math Function1/1 -> Divide/2
  Divide/1 -> Switch/3
  Switch/1 -> Out1/1
  e/1 -> Sign/1, Abs/1, Divide/1
